simulink model "int322416"  (Simulink 7.7)
settings: Solver=FixedStepDiscrete  StartTime=0.0  StopTime=1  RelTol=1e-3
values from neighbouring files (symbols this model uses):
  D = [  1 -1  1 -1  1  1 -1 -1 ... (first row only)    [cdma.m]    (also in compressed_sampling.m = idct(eye(5000,5000)))
libraries: simulink x1, dspsrcs4 x1
settings Model: Creator=ArunKB  LastModifiedBy=ArunKB

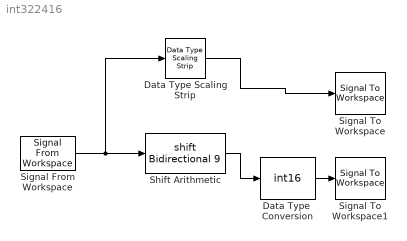
== system int322416 ==
  Data Type Scaling Strip : simulink/Signal Attributes/Data Type Scaling Strip  SystemSampleTime=-1
  Data Type  Conversion : DataTypeConversion  OutDataTypeStr=int16  SaturateOnIntegerOverflow=on  RndMeth=Zero
  Shift Arithmetic : ArithShift  BitShiftNumber=9
  Signal From Workspace : dspsrcs4/Signal From Workspace  SystemSampleTime=-1  X=y  Ts=1  nsamps=1  OutputAfterFinalValue=Setting to zero  ignoreOrWarnInputAndFrameLengths=off
  Signal To Workspace : SignalToWorkspace  VariableName=yout  SaveFormat=Array  Save2DMode=2-D array (concatenate along first dimension)
      settings: CopyFcn=dspblkcopystw(gcbh);
  Signal To Workspace1 : SignalToWorkspace  VariableName=yout1  SaveFormat=Array  Save2DMode=2-D array (concatenate along first dimension)
      settings: CopyFcn=dspblkcopystw(gcbh);
  wires:
  Signal From Workspace/1 -> Shift Arithmetic/1, Data Type Scaling Strip/1
  Data Type Scaling Strip/1 -> Signal To Workspace/1
  Shift Arithmetic/1 -> Data Type  Conversion/1
  Data Type  Conversion/1 -> Signal To Workspace1/1
